simulink model "based_FOC"  (R2024b)
settings: Solver=FixedStepAuto  StartTime=0.0  StopTime=inf  FixedStep=0.000001  MaxStep=1e-6  RelTol=1e-3
undefined symbols (not defined in the file): DiscIntNeverNeededParam, F1, flux, gamma, K1, K2, L, Ld, Lq, Period, PLL_P, Pn, Rs, Ts, U_ref, Udc
libraries: eeGeneralControl x3, spsDCVoltageSourceLib x1, spsGroundLib x1, spsPermanentMagnetSynchronousMachineLib x1, slpidlib x1, simulink x1, spsTwoLevelConverterLib x1, sps_lib x1
settings Model: DataDictionary=Based_FOC_Data.sldd  SimulationMode=rapid-accelerator  Creator=sa127  LastModifiedBy=sa127
settings OptimizationCC: DefaultParameterBehavior=Inlined  UseDivisionForNetSlopeComputation=on  GainParamInheritBuiltInType=on  UseFloatMulNetSlope=on  InlineInvariantSignals=on  PassReuseOutputArgsAs=Individual arguments  ZeroExternalMemoryAtStartup=off  ZeroInternalMemoryAtStartup=off  NoFixptDivByZeroProtection=on  EfficientFloat2IntCast=on  LifeSpan=1  OptimizeBlockOrder=speed  DifferentSizesBufferReuse=on  MultiThreadedLoops=on  EfficientTunableParamExpr=on
settings DebuggingCC: ParamSuppressDoubleToSinglePrecisionLossMsg=on  ParameterTunabilityLossMsg=error
settings HardwareCC: ProdBitPerPointer=32  ProdBitPerSizeT=32  ProdBitPerPtrDiffT=32  ProdLargestAtomicInteger=Long  ProdLargestAtomicFloat=Double  ProdWordSize=32  ProdLongLongMode=on  ProdHWDeviceType=ARM Compatible->ARM Cortex-M
settings SFSimCC: MATLABDynamicMemAlloc=off
settings RTWCC: Description=Embedded Coder  SystemTargetFile=ert.tlc  TemplateMakefile=ert_default_tmf  GenerateReport=on  IncludeHyperlinkInReport=on  LaunchReport=on  GenerateTraceInfo=on  GenerateTraceReport=on  GenerateTraceReportSl=on  GenerateTraceReportSf=on  GenerateTraceReportEml=on  GenerateWebview=on  GenerateCodeMetricsReport=on  GenerateCodeReplacementReport=on
settings CodeAppCC: ForceParamTrailComments=on  IgnoreCustomStorageClasses=off  OperatorAnnotations=on  SimulinkDataObjDesc=on  SFDataObjDesc=on  CustomSymbolStrGlobalVar=rt$N$M  CustomSymbolStrType=$N$M  CustomSymbolStrFcn=$N$M$F  CustomSymbolStrMacro=$N$M  InsertBlockDesc=on
settings ERTTargetCC: TargetLangStandard=C99 (ISO)  CodeReplacementLibrary=ARM Cortex-M  GenerateSampleERTMain=on  IncludeMdlTerminateFcn=off  CombineSignalStateStructs=on  SupportComplex=off  SupportNonInlinedSFcns=on  ERTCustomFileTemplate=example_file_process.tlc  ERTFilePackagingFormat=CompactWithDataFile

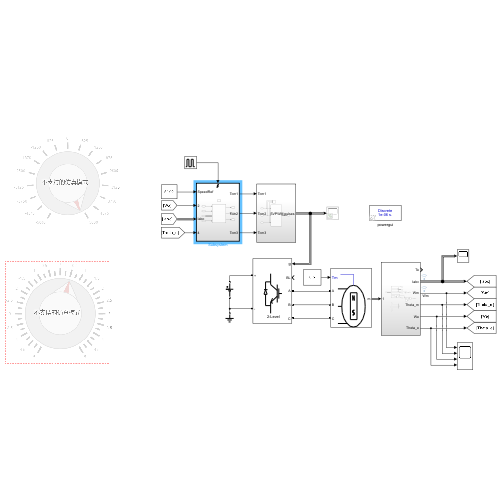
[thumbnail: Simulink's stored preview of the top-level diagram]
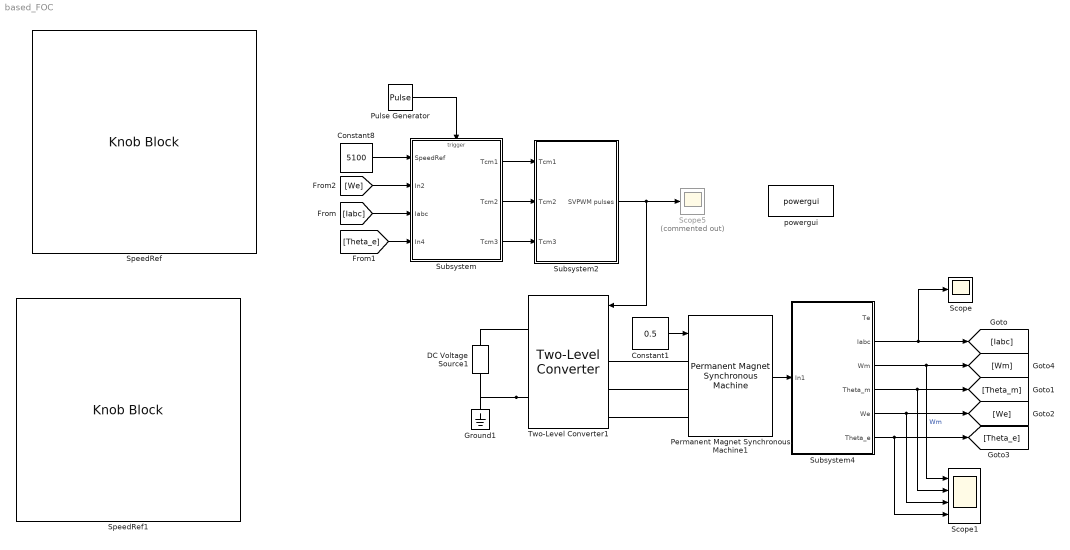
== system based_FOC ==
  Constant1 : Constant  Value=0.5
  Constant8 : Constant  Value=5100
  DC Voltage Source1 : spsDCVoltageSourceLib/DC Voltage Source  Amplitude=300  Measurements=None
  Ground1 : spsGroundLib/Ground  LConnTagsString=a
  Permanent Magnet Synchronous Machine1 : spsPermanentMagnetSynchronousMachineLib/Permanent Magnet Synchronous Machine  NbPhases=3  FluxDistribution=Sinusoidal  RotorType=Salient-pole  MechanicalLoad=Torque Tm  PresetModel="04:  6 Nm 300 Vdc 4500 RPM - 6 Nm"  ShowDetailedParameters=on  MeasurementBus=on  Resistance=0.62  Inductance=8.5e-3  dqInductances=[0.001971 0.002179]  La=0.002075  MachineConstant=Flux linkage established by magnets (V.s)  Flux=0.08627  VoltageCst=62.5906  TorqueCst=0.51762  Flat=120  Mechanical=[0.0003617 9.444e-05 4 0]  PolePairs=4  InitialConditions=[0,0, 0,0]  InitialConditions5ph=[0 0 0 0 0 0]  RefAngle=Aligned with phase A axis (original Park)  IterativeDiscreteModel=Trapezoidal non iterative  TsBlock=-1  TsPowergui=0
  Pulse Generator : DiscretePulseGenerator  PulseType=Time based  Period=0.0001  PulseWidth=50
  Scope : Scope
  Scope1 : Scope  NumInputPorts=4
  Scope5 : Scope  Commented=on
  SpeedRef : KnobBlock  ScaleMin=-5000  ScaleMax=5000
  SpeedRef1 : KnobBlock  ScaleMin=-5  ScaleMax=5
  Subsystem : Subsystem
  Subsystem2 : Subsystem
  Subsystem4 : Subsystem
  Two-Level Converter1 : spsTwoLevelConverterLib/Two-Level Converter  ModelType=Switching function  Ron=1e-3  Rs=1e6  Cs=inf  Vforward=[0,0]  Ron_Diode=1e-3  Rs_Diode=1e6  Cs_Diode=inf  Vf_Diode=1e-3  Rs_CurrentSource=inf  Ron_ACsource=1e-3
      settings: LibrarySourceBlock=sps_lib/Power Electronics/Two-Level Converter
  powergui : sps_lib/powergui  Priority=1  SimulationMode=Discrete  SampleTime=0.000001  frequency=60  Iterations=50  frequencyindice=0  Pbase=100e6  ErrMax=1e-4  UnitsV=kV  UnitsW=MW  buscounter=0  FunctionMessages=off  echomessages=off  EnableUseOfTLC=off  CurrentSourceSwitches=off  DisableSnubberDevices=off  DisableRonSwitches=off  DisableVfSwitches=off  DisplayEquations=off  AutomaticDiscreteSolvers=off  SolverType=Tustin/Backward Euler (TBE)  Interpol=off  ExternalGateDelay=off  methode=off  Ts=100  x0status=blocks  SPID=on  SwTol=0  HookPort=off  NonlinearTolerance=1e-4  nMaxIteration=100  ContinueOnMaxIteration=off  RestoreLinks=warning  ResistiveCurrentMeasurement=off  Frange=[0:2:500]  Ylog=off  Xlog=on  ShowGrid=off  save=off  variable=ZData  structure=0  ZoomFFT=off  StartTime=0.0  cycles=1  DisplayStyle=1  fundamental=60  FreqAxis=off  MaxFrequency=1000  frequencyindicesteady=1  RmsSteady=1  display=off
  wires:
  Permanent Magnet Synchronous Machine1/1 -> Subsystem4/1(In1)
  Subsystem4/2(Iabc) -> Scope/1, [Iabc]
  Subsystem4/3(Wm) -> Scope1/1, [Wm]  "Wm"
  Subsystem4/4(Theta_m) -> [Theta_m], Scope1/2
  Subsystem4/5(We) -> Scope1/3, [We]
  Subsystem4/6(Theta_e) -> Scope1/4, [Theta_e]
  Subsystem2/1(SVPWM pulses) -> Two-Level Converter1/1, Scope5/1
  Constant1/1 -> Permanent Magnet Synchronous Machine1/1
  Constant8/1 -> Subsystem/1(SpeedRef)
  [We] -> Subsystem/2(In2)
  [Iabc] -> Subsystem/3(Iabc)
  [Theta_e] -> Subsystem/4(In4)
  Subsystem/1(Tcm1) -> Subsystem2/1(Tcm1)
  Subsystem/2(Tcm2) -> Subsystem2/2(Tcm2)
  Subsystem/3(Tcm3) -> Subsystem2/3(Tcm3)
  Pulse Generator/1 -> Subsystem/Trigger
  connections:
  Two-Level Converter1/RConn2 -- DC Voltage Source1/LConn1 -- Ground1/LConn1
  Two-Level Converter1/LConn2 -- Permanent Magnet Synchronous Machine1/LConn2
  Two-Level Converter1/LConn1 -- Permanent Magnet Synchronous Machine1/LConn1
  Two-Level Converter1/LConn3 -- Permanent Magnet Synchronous Machine1/LConn3
  DC Voltage Source1/RConn1 -- Two-Level Converter1/RConn1

== system based_FOC/Subsystem ==
  SpeedRef : Inport
  In2 : Inport  Port=2
  Iabc : Inport  Port=3
  In4 : Inport  Port=4
  Trigger : TriggerPort  VariantControl=(inherit)  PortDimensions=1
  Sensorless : Subsystem
  Tcm1 : Outport
  Tcm2 : Outport  Port=2
  Tcm3 : Outport  Port=3
  wires:
  Sensorless/2(Tcm2) -> Tcm2/1
  SpeedRef/1 -> Sensorless/1(SpeedRef)
  In2/1 -> Sensorless/2(In2)
  In4/1 -> Sensorless/4(In4)
  Iabc/1 -> Sensorless/3(Iabc)
  Sensorless/3(Tcm3) -> Tcm3/1
  Sensorless/1(Tcm1) -> Tcm1/1

== system based_FOC/Subsystem2 ==
  Tcm1 : Inport
  Tcm2 : Inport  Port=2
  Tcm3 : Inport  Port=3
  Scope1 : Scope  NumInputPorts=3
  Subsystem1 : Subsystem
  SVPWM pulses : Outport
  wires:
  Tcm1/1 -> Subsystem1/1(Tcm1), Scope1/1
  Tcm2/1 -> Subsystem1/2(Tcm2), Scope1/2
  Tcm3/1 -> Subsystem1/3(Tcm3), Scope1/3
  Subsystem1/1(SVPWM pulses) -> SVPWM pulses/1

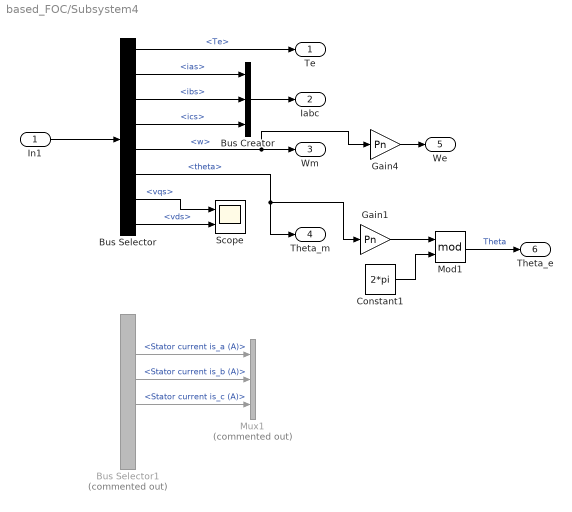
== system based_FOC/Subsystem4 ==
  In1 : Inport
  Bus Creator : BusCreator  Inputs=3
  Bus Selector : BusSelector  OutputSignals=Te,ias,ibs,ics,w,theta,vqs,vds
  Bus Selector1 : BusSelector  Commented=on  OutputSignals=Electromagnetic torque Te (N*m),Stator current is_a (A),Stator current is_b (A),Stator current is_c (A),Rotor speed wm (rad/s),Rotor angle thetam (rad)
  Constant1 : Constant  Value=2*pi
  Gain1 : Gain  Gain=Pn
  Gain4 : Gain  Gain=Pn
  Mod1 : Math  Operator=mod
  Mux1 : Mux  Commented=on  Inputs=3
  Scope : Scope  NumInputPorts=2
  Te : Outport
  Iabc : Outport  Port=2
  Wm : Outport  Port=3
  Theta_m : Outport  Port=4
  We : Outport  Port=5
  Theta_e : Outport  Port=6
  wires:
  Bus Selector/2 -> Bus Creator/1  "<ias>"
  Bus Selector/4 -> Bus Creator/3  "<ics>"
  Bus Selector/3 -> Bus Creator/2  "<ibs>"
  Bus Selector1/4 -> Mux1/3  "<Stator current is_c (A)>"
  Bus Selector1/3 -> Mux1/2  "<Stator current is_b (A)>"
  Bus Selector1/2 -> Mux1/1  "<Stator current is_a (A)>"
  In1/1 -> Bus Selector/1
  Bus Selector/1 -> Te/1  "<Te>"
  Bus Selector/5 -> Gain4/1, Wm/1  "<w>"
  Bus Selector/6 -> Gain1/1, Theta_m/1  "<theta>"
  Bus Selector/8 -> Scope/2  "<vds>"
  Bus Selector/7 -> Scope/1  "<vqs>"
  Constant1/1 -> Mod1/2
  Gain1/1 -> Mod1/1
  Gain4/1 -> We/1
  Mod1/1 -> Theta_e/1  "Theta"
  Bus Creator/1 -> Iabc/1

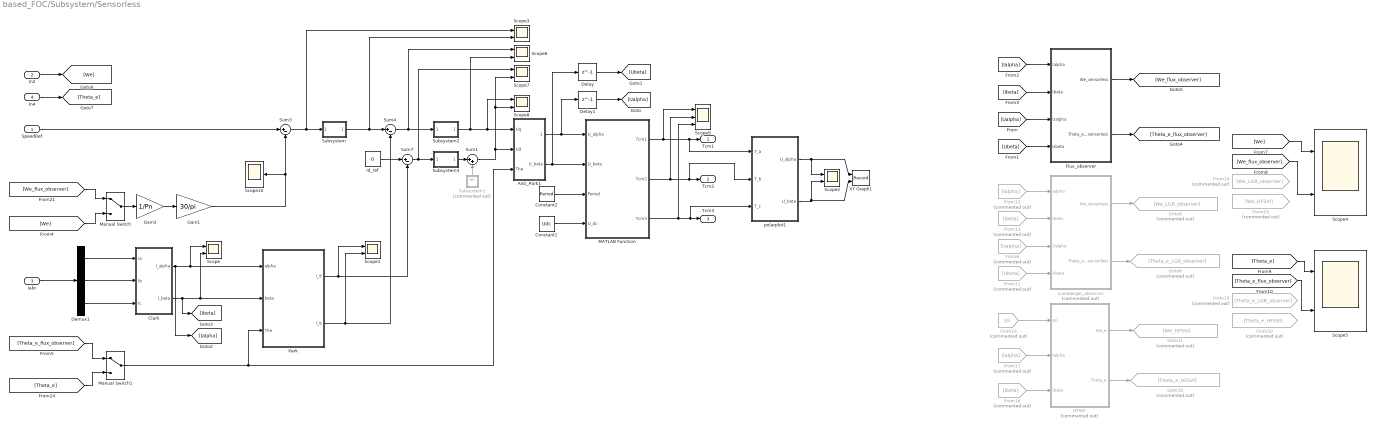
== system based_FOC/Subsystem/Sensorless ==
  SpeedRef : Inport
  In2 : Inport  Port=2
  Iabc : Inport  Port=3
  In4 : Inport  Port=4
  Anti_Park1 : Subsystem
  Clark : Subsystem
  Constant1 : Constant  Value=Udc
  Constant2 : Constant  Value=Period
  Delay : Delay  DelayLength=1
  Delay1 : Delay  DelayLength=1
  Demux1 : Demux  Outputs=3
  Flux_observer : Subsystem  TreatAsAtomicUnit=on
  From11 : From  Commented=on  GotoTag=Ubeta
  From12 : From  Commented=on  GotoTag=Ialpha
  From13 : From  Commented=on  GotoTag=Ibeta
  From14 : From  Commented=on  GotoTag=We_LGB_observer
  From15 : From  Commented=on  GotoTag=Theta_e_LGB_observer
  From16 : From  Commented=on  GotoTag=Uh  TagVisibility=global
  From17 : From  Commented=on  GotoTag=Ialpha
  From18 : From  Commented=on  GotoTag=Ibeta
  From19 : From  Commented=on  GotoTag=We_HFSVI
  From20 : From  Commented=on  GotoTag=Theta_e_HFSVI
  From6 : From  Commented=on  GotoTag=Ualpha
  Gain1 : Gain  Gain=30/pi
  Gain3 : Gain  Gain=1/Pn
  Goto10 : Goto  Commented=on  GotoTag=Theta_e_HFSVI
  Goto11 : Goto  Commented=on  GotoTag=We_HFSVI
  Goto8 : Goto  Commented=on  GotoTag=Theta_e_LGB_observer
  Goto9 : Goto  Commented=on  GotoTag=We_LGB_observer
  HFSVI : Subsystem  Commented=on
  Id_ref : Constant  Value=0
  Luenberger_observer : Subsystem  Commented=on  TreatAsAtomicUnit=on
  MATLAB Function : MATLAB Function  TreatAsAtomicUnit=on
  Manual Switch : ManualSwitch
  Manual Switch1 : ManualSwitch
  Park : Subsystem
  Scope{,1..8} (9 alike) : Scope  NumInputPorts=2
  Scope10 : Scope
  Scope9 : Scope  NumInputPorts=3
  Subsystem : Subsystem  mask{Kp=0.001, Ki=0.004, Kd=0, Ts=0.0001, max_Integral=500, min_Integral=-500, max_output=500, min_output=-500}
      mask prompts: max_Integral "积分上限"; min_Integral "积分下限"; max_output "输出上限"; min_output "输出下限"
      mask DialogControl DescTextVar Prompt: PID控制器
      mask DialogControl ParameterGroupVar Prompt: 参数
      mask Display: fprintf('MyPID');
  Subsystem1 : Subsystem  Commented=on
  Subsystem2 : Subsystem  mask{Kp=20, Ki=3000, Kd=0, Ts=0.0001, max_Integral=500, min_Integral=-500, max_output=500, min_output=-500}
      mask prompts: max_Integral "积分上限"; min_Integral "积分下限"; max_output "输出上限"; min_output "输出下限"
      mask DialogControl DescTextVar Prompt: PID控制器
      mask DialogControl ParameterGroupVar Prompt: 参数
      mask Display: fprintf('MyPID');
  Subsystem3 : Subsystem  mask{Kp=20, Ki=3000, Kd=0, Ts=0.0001, max_Integral=500, min_Integral=-500, max_output=500, min_output=-500}
      mask prompts: max_Integral "积分上限"; min_Integral "积分下限"; max_output "输出上限"; min_output "输出下限"
      mask DialogControl DescTextVar Prompt: PID控制器
      mask DialogControl ParameterGroupVar Prompt: 参数
      mask Display: fprintf('MyPID');
  Sum1 : Sum  Inputs=|++
  Sum3 : Sum  Inputs=|+-
  Sum4 : Sum  Inputs=|+-
  Sum7 : Sum  Inputs=|+-
  XY Graph1 : Record  FileSettingsInternal="{\"entries\":[{\"content\":{\"excelSettings\":{\"content\":{},\"type\":\"Streamout.ExcelSettings\"}},\"type\":\"Streamout.FileSettingStorage\",\"uuid\":\"\"}],\"packageUris\":[\"http:\\/\\/schema.mathworks.com\\/mf0\\/streamout_blocks\\/R2020a\"],\"version\":\"1.0\"}"  Layout=[1 1]  SignalsInternal="{\"entries\":[{\"content\":{\"signals\":[{\"content\":{\"blockPath\":[],\"dimensions\":[1],\"domain\":\"\",\"lineColor\":\"#ff6929\",\"plots\":[ 1 ],\"port\":1,\"sid\":[\"\"],\"signalID\":1,\"signalName\":\"polarplot1:1\"},\"type\":\"RecordBlkView.Signal\",\"uuid\":\"\"},{\"content\":{\"blockPath\":[],\"dimensions\":[1],\"domain\":\"\",\"lineColor\":\"#b746ff\",\"plots\":[ 1 ],\"port\":2,\"sid\":[\"\"],\"signalID\":2,\"signalName\":\"polarplot1:2\"},\"type\":\"RecordBlkView.Signal\",\"uuid\":\"\"}]},\"type\":\"RecordBlkView.InputSignals\",\"uuid\":\"\"}],\"packageUris\":[\"http:\\/\\/schema.mathworks.com\\/mf0\\/streamout_blocks\\/R2020a\"],\"version\":\"1.0\"}"  VisualizationBindings="{\"xyplotplugin\":{\"info\":[{\"series\":[{\"bindingParametersList\":[{\"parameter\":\"X-Axis\",\"signalID\":1,\"signalName\":\"polarplot1:1\"},{\"parameter\":\"Y-Axis\",\"signalID\":2,\"signalName\":\"polarplot1:2\"},{\"parameter\":\"X-Axis\",\"signalID\":1,\"signalName\":\"polarplot1:1\"},{\"parameter\":\"Y-Axis\",\"signalID\":2,\"signalName\":\"polarplot1:2\"}],\"seriesID\":0}],\"subplotID\":1}]}}"  CompatibilityTag=XY
  polarplot1 : MATLAB Function  TreatAsAtomicUnit=on
  Tcm1 : Outport
  Tcm2 : Outport  Port=2
  Tcm3 : Outport  Port=3
  wires:
  Park/1(I_d) -> Scope1/1, Sum7/2
  Sum7/1 -> Scope7/1, Subsystem3/1(error)
  Gain1/1 -> Sum3/2, Scope10/1
  Demux1/3 -> Clark/3(Ic)
  Demux1/1 -> Clark/1(Ia)
  Iabc/1 -> Demux1/1
  Clark/1(I_alpha) -> [Ialpha], Scope/1, Park/1(alpha)
  Clark/2(I_beta) -> [Ibeta], Scope/2, Park/2(beta)
  Id_ref/1 -> Sum7/1
  Sum3/1 -> Scope3/1, Subsystem/1(error)
  Park/2(I_q) -> Scope1/2, Sum4/2
  Sum4/1 -> Scope6/1, Subsystem2/1(error)
  Demux1/2 -> Clark/2(Ib)
  Gain3/1 -> Gain1/1
  SpeedRef/1 -> Sum3/1
  Anti_Park1/2(U_beta) -> MATLAB Function/2(U_beta), Delay/1
  Subsystem2/1(output) -> Scope6/2, Anti_Park1/1(Uq), Scope8/1
  Manual Switch1/1 -> Anti_Park1/3(The), Park/3(The)
  [We] -> Scope4/1
  [Theta_e] -> Scope5/1
  Delay/1 -> [Ubeta]
  Delay1/1 -> [Ualpha]
  [Ialpha] -> Flux_observer/1(Ialpha)
  [Ibeta] -> Flux_observer/2(Ibeta)
  [Ualpha] -> Flux_observer/3(Ualpha)
  [Ubeta] -> Flux_observer/4(Ubeta)
  Flux_observer/2(Theta_e_sensorless) -> [Theta_e_flux_observer]
  Flux_observer/1(We_sensorless) -> [We_flux_observer]
  In2/1 -> [We]
  In4/1 -> [Theta_e]
  From12/1 -> Luenberger_observer/1(Ialpha)
  From13/1 -> Luenberger_observer/2(Ibeta)
  From6/1 -> Luenberger_observer/3(Ualpha)
  From11/1 -> Luenberger_observer/4(Ubeta)
  Luenberger_observer/1(We_sensorless) -> Goto9/1
  Luenberger_observer/2(Theta_e_sensorless) -> Goto8/1
  Subsystem/1(output) -> Scope3/2, Sum4/1
  Subsystem3/1(output) -> Sum1/1
  Sum1/1 -> Anti_Park1/2(Ud), Scope8/2, Scope7/2
  From16/1 -> HFSVI/1(Uh)
  From17/1 -> HFSVI/2(Ialpha)
  From18/1 -> HFSVI/3(Ibeta)
  HFSVI/2(Theta_e) -> Goto10/1
  HFSVI/1(We_e) -> Goto11/1
  Manual Switch/1 -> Gain3/1
  [We] -> Manual Switch/2
  [We_flux_observer] -> Manual Switch/1
  [Theta_e] -> Manual Switch1/2
  [Theta_e_flux_observer] -> Manual Switch1/1
  Subsystem1/1(Uh) -> Sum1/2
  [We_flux_observer] -> Scope4/2
  [Theta_e_flux_observer] -> Scope5/2
  Anti_Park1/1(U_alpha) -> MATLAB Function/1(U_alpha), Delay1/1
  Constant2/1 -> MATLAB Function/3(Period)
  Constant1/1 -> MATLAB Function/4(U_dc)
  MATLAB Function/1(Tcm1) -> polarplot1/1(T_a), Tcm1/1, Scope9/1
  MATLAB Function/2(Tcm2) -> polarplot1/2(T_b), Tcm2/1, Scope9/2
  MATLAB Function/3(Tcm3) -> polarplot1/3(T_c), Tcm3/1, Scope9/3
  polarplot1/1(U_alpha) -> XY Graph1/1, Scope2/1
  polarplot1/2(U_beta) -> XY Graph1/2, Scope2/2

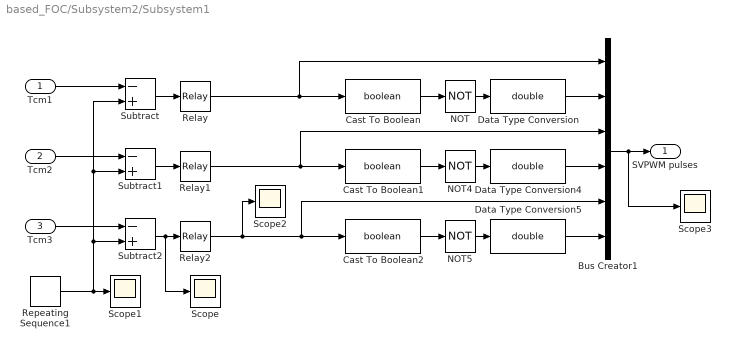
== system based_FOC/Subsystem2/Subsystem1 ==
  Tcm1 : Inport
  Tcm2 : Inport  Port=2
  Tcm3 : Inport  Port=3
  Bus Creator1 : BusCreator  Inputs=6
  Cast To Boolean : DataTypeConversion  OutDataTypeStr=boolean  SaturateOnIntegerOverflow=off  RndMeth=Floor
  Cast To Boolean1 : DataTypeConversion  OutDataTypeStr=boolean  SaturateOnIntegerOverflow=off  RndMeth=Floor
  Cast To Boolean2 : DataTypeConversion  OutDataTypeStr=boolean  SaturateOnIntegerOverflow=off  RndMeth=Floor
  Data Type Conversion : DataTypeConversion  OutDataTypeStr=double  SaturateOnIntegerOverflow=off  RndMeth=Floor
  Data Type Conversion4 : DataTypeConversion  OutDataTypeStr=double  SaturateOnIntegerOverflow=off  RndMeth=Floor
  Data Type Conversion5 : DataTypeConversion  OutDataTypeStr=double  SaturateOnIntegerOverflow=off  RndMeth=Floor
  NOT : Logic  Operator=NOT  IconShape=distinctive  AllPortsSameDT=off  OutDataTypeStr=boolean
  NOT4 : Logic  Operator=NOT  IconShape=distinctive  AllPortsSameDT=off  OutDataTypeStr=boolean
  NOT5 : Logic  Operator=NOT  IconShape=distinctive  AllPortsSameDT=off  OutDataTypeStr=boolean
  Relay : Relay
  Relay1 : Relay
  Relay2 : Relay
  Repeating Sequence1 : simulink/Sources/Repeating Sequence  rep_seq_t=[0 Ts/2 Ts]  rep_seq_y=[0 Period/2 0]
  Scope{,1..3} (4 alike) : Scope
  Subtract : Sum  Inputs=-+
  Subtract1 : Sum  Inputs=-+
  Subtract2 : Sum  Inputs=-+
  SVPWM pulses : Outport
  wires:
  Tcm3/1 -> Subtract2/1
  Cast To Boolean/1 -> NOT/1
  Subtract/1 -> Relay/1
  Relay2/1 -> Scope2/1, Bus Creator1/5, Cast To Boolean2/1
  Subtract2/1 -> Scope/1, Relay2/1
  Cast To Boolean2/1 -> NOT5/1
  Subtract1/1 -> Relay1/1
  Repeating Sequence1/1 -> Subtract2/2, Subtract1/2, Subtract/2, Scope1/1
  Tcm1/1 -> Subtract/1
  NOT/1 -> Data Type Conversion/1
  Cast To Boolean1/1 -> NOT4/1
  Bus Creator1/1 -> Scope3/1, SVPWM pulses/1
  NOT5/1 -> Data Type Conversion5/1
  Relay1/1 -> Bus Creator1/3, Cast To Boolean1/1
  Relay/1 -> Bus Creator1/1, Cast To Boolean/1
  Tcm2/1 -> Subtract1/1
  Data Type Conversion5/1 -> Bus Creator1/6
  Data Type Conversion/1 -> Bus Creator1/2
  NOT4/1 -> Data Type Conversion4/1
  Data Type Conversion4/1 -> Bus Creator1/4

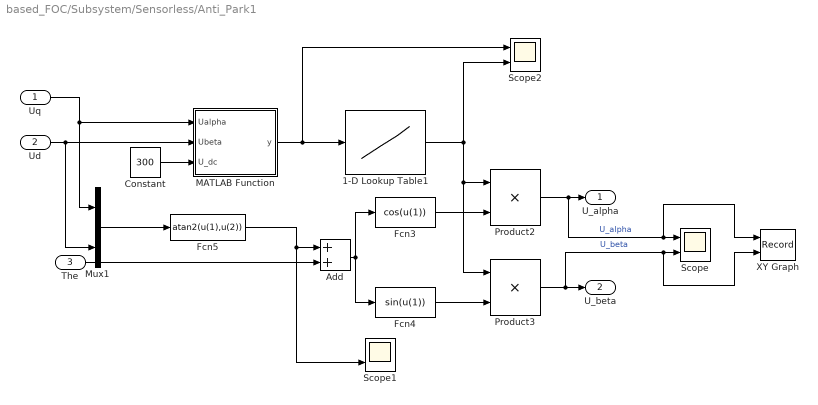
== system based_FOC/Subsystem/Sensorless/Anti_Park1 ==
  Uq : Inport
  Ud : Inport  Port=2
  The : Inport  Port=3
  1-D Lookup Table1 : Lookup_n-D  NumberOfTableDimensions=1  BreakpointsForDimension1=F1  Table=U_ref  ExtrapMethod=Clip  UseLastTableValue=on  InternalRulePriority=Speed  RndMeth=Simplest
  Add : Sum
  Constant : Constant  Value=300
  Fcn3 : Fcn  Expr=cos(u(1))
  Fcn4 : Fcn  Expr=sin(u(1))
  Fcn5 : Fcn  Expr=atan2(u(1),u(2))
  MATLAB Function : MATLAB Function  TreatAsAtomicUnit=on
  Mux1 : Mux  Inputs=2
  Product2 : Product
  Product3 : Product
  Scope : Scope  NumInputPorts=2
  Scope1 : Scope  NumInputPorts=2
  Scope2 : Scope  NumInputPorts=2
  XY Graph : Record  FileSettingsInternal="{\"entries\":[{\"content\":{\"excelSettings\":{\"content\":{},\"type\":\"Streamout.ExcelSettings\"}},\"type\":\"Streamout.FileSettingStorage\",\"uuid\":\"\"}],\"packageUris\":[\"http:\\/\\/schema.mathworks.com\\/mf0\\/streamout_blocks\\/R2020a\"],\"version\":\"1.0\"}"  Layout=[1 1]  SignalsInternal="{\"entries\":[{\"content\":{\"signals\":[{\"content\":{\"blockPath\":[],\"dimensions\":[1],\"domain\":\"\",\"lineColor\":\"#139fff\",\"lineWidth\":2,\"plots\":[ 1 ],\"port\":1,\"sid\":[\"\"],\"signalID\":1,\"signalName\":\"U_alpha\"},\"type\":\"RecordBlkView.Signal\",\"uuid\":\"\"},{\"content\":{\"blockPath\":[],\"dimensions\":[1],\"domain\":\"\",\"lineColor\":\"#22b573\",\"lineWidth\":2,\"plots\":[ 1 ],\"port\":2,\"sid\":[\"\"],\"signalID\":2,\"signalName\":\"U_beta\"},\"type\":\"RecordBlkView.Signal\",\"uuid\":\"\"}]},\"type\":\"RecordBlkView.InputSignals\",\"uuid\":\"\"}],\"packageUris\":[\"http:\\/\\/schema.mathworks.com\\/mf0\\/streamout_blocks\\/R2020a\"],\"version\":\"1.0\"}"  VisualizationBindings="{\"xyplotplugin\":{\"info\":[{\"series\":[{\"bindingParametersList\":[{\"parameter\":\"X-Axis\",\"signalID\":1,\"signalName\":\"U_alpha\"},{\"parameter\":\"Y-Axis\",\"signalID\":2,\"signalName\":\"U_beta\"},{\"parameter\":\"X-Axis\",\"signalID\":1,\"signalName\":\"U_alpha\"},{\"parameter\":\"Y-Axis\",\"signalID\":2,\"signalName\":\"U_beta\"}],\"seriesID\":0}],\"subplotID\":1}]}}"  CompatibilityTag=XY
  U_alpha : Outport
  U_beta : Outport  Port=2
  wires:
  Fcn5/1 -> Scope1/2, Add/1
  Ud/1 -> MATLAB Function/2(Ubeta), Mux1/2
  Fcn3/1 -> Product2/2
  Fcn4/1 -> Product3/2
  Mux1/1 -> Fcn5/1
  1-D Lookup Table1/1 -> Scope2/2, Product2/1, Product3/1
  Product2/1 -> XY Graph/1, Scope/1, U_alpha/1  "U_alpha"
  Product3/1 -> XY Graph/2, Scope/2, U_beta/1  "U_beta"
  The/1 -> Add/2
  Add/1 -> Fcn3/1, Fcn4/1
  Constant/1 -> MATLAB Function/3(U_dc)
  Uq/1 -> MATLAB Function/1(Ualpha), Mux1/1
  MATLAB Function/1(y) -> 1-D Lookup Table1/1, Scope2/1

== system based_FOC/Subsystem/Sensorless/Clark ==
  Ia : Inport
  Ib : Inport  Port=2
  Ic : Inport  Port=3
  Fcn : Fcn  Expr=(u(1)-0.5*u(2)-0.5*u(3))*2/3
  Fcn1 : Fcn  Expr=(sqrt(3)/2*u(2)-sqrt(3)/2*u(3))*2/3
  Mux : Mux  Inputs=3
  I_alpha : Outport
  I_beta : Outport  Port=2
  wires:
  Ib/1 -> Mux/2
  Fcn1/1 -> I_beta/1
  Ic/1 -> Mux/3
  Mux/1 -> Fcn1/1, Fcn/1
  Fcn/1 -> I_alpha/1
  Ia/1 -> Mux/1

== system based_FOC/Subsystem/Sensorless/Flux_observer ==
  Ialpha : Inport
  Ibeta : Inport  Port=2
  Ualpha : Inport  Port=3
  Ubeta : Inport  Port=4
  OBSERVER : Subsystem
  PLL : Subsystem
  Scope : Scope  NumInputPorts=2
  We_sensorless : Outport
  Theta_e_sensorless : Outport  Port=2
  wires:
  Ibeta/1 -> OBSERVER/2(Ibeta)
  OBSERVER/1(sin) -> Scope/1, PLL/1(sin)  "sin_theta"
  OBSERVER/2(cos) -> Scope/2, PLL/2(cos)  "cos_theta"
  PLL/1(We) -> We_sensorless/1
  PLL/2(Theta_e) -> Theta_e_sensorless/1
  Ualpha/1 -> OBSERVER/3(Ualpha)
  Ubeta/1 -> OBSERVER/4(Ubeta)
  Ialpha/1 -> OBSERVER/1(Ialpha)

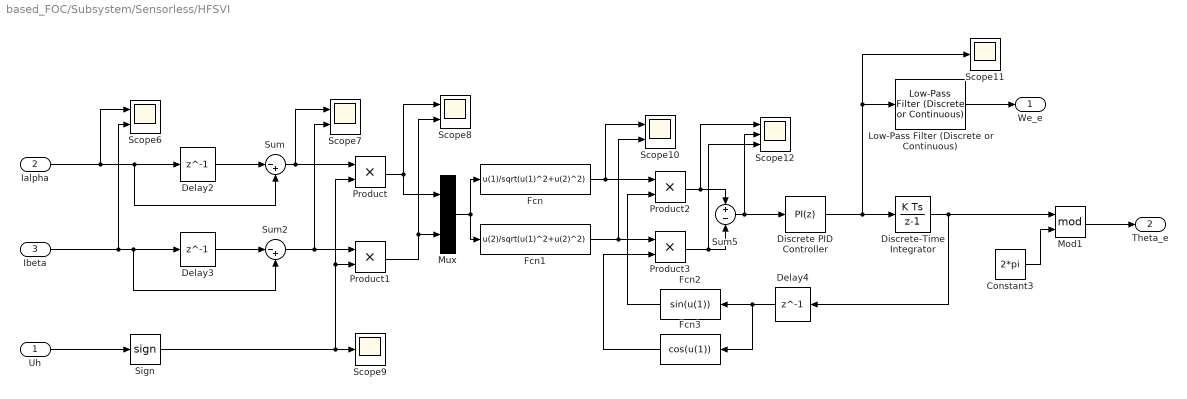
== system based_FOC/Subsystem/Sensorless/HFSVI ==
  Uh : Inport
  Ialpha : Inport  Port=2
  Ibeta : Inport  Port=3
  Constant3 : Constant  Value=2*pi
  Delay2 : Delay  DelayLength=1  InitialCondition=0
  Delay3 : Delay  DelayLength=1  InitialCondition=0
  Delay4 : Delay  DelayLength=1  InitialCondition=0
  Discrete PID Controller : slpidlib/PID Controller  Controller=PI  Form=Parallel  TimeDomain=Discrete-time  UseExternalTs=off  SampleTime=-1  IntegratorMethod=Forward Euler  FilterMethod=Forward Euler  ControllerParametersSource=internal  P=400  I=40000  UseKiTs=off  D=0  UseExternalDerivativeSource=off  N=100  UseFilter=on  TunerSelectOption=Transfer Function Based (PID Tuner App)  InitialConditionSource=internal  InitialConditionForIntegrator=0  InitialConditionForFilter=0  DifferentiatorICPrevScaledInput=0  ExternalReset=none  TrackingMode=off  Kt=1  LimitOutput=off  SatLimitsSource=internal  UpperSaturationLimit=inf  LowerSaturationLimit=-inf  LinearizeAsGain=off  AntiWindupMode=none  Kb=1  LimitIntegrator=off  UpperIntegratorSaturationLimit=inf  LowerIntegratorSaturationLimit=-inf  POutMin=[]  POutMax=[]  IOutMin=[]  IOutMax=[]  DOutMin=[]  DOutMax=[]  NOutMin=[]  NOutMax=[]  SumOutMin=[]  SumOutMax=[]  SaturationOutMin=[]  SaturationOutMax=[]  PParamMin=[]  PParamMax=[]  IParamMin=[]  IParamMax=[]  DParamMin=[]  DParamMax=[]  NParamMin=[]  NParamMax=[]  KbParamMin=[]  KbParamMax=[]  KtParamMin=[]  KtParamMax=[]  KbOutMin=[]  KbOutMax=[]  KtOutMin=[]  KtOutMax=[]  IntegratorOutMin=[]  IntegratorOutMax=[]  FilterOutMin=[]  FilterOutMax=[]  SumI1OutMin=[]  SumI1OutMax=[]  SumI2OutMin=[]  SumI2OutMax=[]  SumI3OutMin=[]  SumI3OutMax=[]  SumI4OutMin=[]  SumI4OutMax=[]  SumDOutMin=[]  SumDOutMax=[]  DifferentiatorOutMin=[]  DifferentiatorOutMax=[]  FilterDiffOutCoefMin=[]  FilterDiffOutCoefMax=[]  ReciprocalOutMin=[]  ReciprocalOutMax=[]  SumDenOutMin=[]  SumDenOutMax=[]  SumNumOutMin=[]  SumNumOutMax=[]  DivideOutMin=[]  DivideOutMax=[]  UdiffTsProdOutMin=[]  UdiffTsProdOutMax=[]  NTsProdOutMin=[]  NTsProdOutMax=[]  UintegralTsProdOutMin=[]  UintegralTsProdOutMax=[]  UngainTsProdOutMin=[]  UngainTsProdOutMax=[]  ClampingZeroOutDataTypeStr=Inherit: Inherit via back propagation  ClampingZeroOutMin=[]  ClampingZeroOutMax=[]  FilterDenConstantOutDataTypeStr=Inherit: Inherit via back propagation  FilterDenConstantOutMin=[]  FilterDenConstantOutMax=[]  PCopyOutDataTypeStr=Inherit: Inherit via back propagation  PCopyOutMin=[]  PCopyOutMax=[]  NCopyOutDataTypeStr=Inherit: Inherit via back propagation  NCopyOutMin=[]  NCopyOutMax=[]  IntegratorContinuousStateAttributes=''  IntegratorStateMustResolveToSignalObject=off  IntegratorRTWStateStorageClass=Auto  FilterContinuousStateAttributes=''  FilterStateMustResolveToSignalObject=off  FilterRTWStateStorageClass=Auto  ParallelPVariant=InternalParameters  IdealPVariant=Disabled  IVariant=InternalParameters  DVariant=Disabled  IntegratorVariant=Discrete  SatVariant=Disabled  AWVariant=Passthrough  PCopyVariant=Disabled  TRVariant=Disabled  FdbkBlocksVariant=Forward  IdealPFdbkVariant=Disabled  SatFdbkVariant=Disabled  DerivativeFilterVariant=Disabled  NVariant=Disabled  NCopyVariant=Disabled_SignalSpec  FilterICVariant=Disabled  IntegratorICVariant=InternalICs  ExternalResetVariant=Disabled  TRSumVariant=Passthrough  SumFdbkVariant=Disabled  SumVariant=Sum_PI  TsampFilterVariant=InternalTs  TsampNgainVariant=Passthrough  TsampIntegralVariant=Disabled_SignalSpec  ExternalSaturationOutDataTypeStr=Inherit: Same as second input  DerivativeSourceVariant=Disabled  PreIntVariant=InternalPreInt
  Discrete-Time Integrator : DiscreteIntegrator  SampleTime=-1  ICPrevOutput=DiscIntNeverNeededParam  ICPrevScaledInput=DiscIntNeverNeededParam
  Fcn : Fcn  Expr=u(1)/sqrt(u(1)^2+u(2)^2)
  Fcn1 : Fcn  Expr=u(2)/sqrt(u(1)^2+u(2)^2)
  Fcn2 : Fcn  Expr=sin(u(1))
  Fcn3 : Fcn  Expr=cos(u(1))
  Low-Pass Filter (Discrete or Continuous) : eeGeneralControl/Low-Pass Filter (Discrete or Continuous)  K=1  T=0.02  B=inf  A=-inf  init_option=Inherited from block input  x0=0  Ts=-1
  Mod1 : Math  Operator=mod
  Mux : Mux  Inputs=2
  Product{,1..3} (4 alike) : Product
  Scope{6..8,10} (4 alike) : Scope  NumInputPorts=2
  Scope11 : Scope
  Scope12 : Scope  NumInputPorts=3
  Scope9 : Scope
  Sign : Signum
  Sum : Sum  Inputs=|-+
  Sum2 : Sum  Inputs=|-+
  Sum5 : Sum  Inputs=+-
  We_e : Outport
  Theta_e : Outport  Port=2
  wires:
  Sum2/1 -> Scope7/2, Product1/1
  Ibeta/1 -> Delay3/1, Sum2/2, Scope6/2
  Discrete-Time Integrator/1 -> Delay4/1, Mod1/1
  Product2/1 -> Sum5/1, Scope12/1
  Discrete PID Controller/1 -> Discrete-Time Integrator/1, Scope11/1, Low-Pass Filter (Discrete or Continuous)/1
  Uh/1 -> Sign/1
  Fcn1/1 -> Product3/1, Scope10/2
  Mux/1 -> Fcn/1, Fcn1/1
  Product/1 -> Scope8/1, Mux/1
  Sum/1 -> Scope7/1, Product/1
  Product3/1 -> Scope12/3, Sum5/2
  Delay4/1 -> Fcn2/1, Fcn3/1
  Product1/1 -> Scope8/2, Mux/2
  Ialpha/1 -> Scope6/1, Delay2/1, Sum/2
  Low-Pass Filter (Discrete or Continuous)/1 -> We_e/1
  Delay3/1 -> Sum2/1
  Sum5/1 -> Discrete PID Controller/1, Scope12/2
  Sign/1 -> Product/2, Product1/2, Scope9/1
  Delay2/1 -> Sum/1
  Fcn2/1 -> Product2/2
  Fcn3/1 -> Product3/2
  Fcn/1 -> Scope10/1, Product2/1
  Constant3/1 -> Mod1/2
  Mod1/1 -> Theta_e/1

== system based_FOC/Subsystem/Sensorless/Luenberger_observer ==
  Ialpha : Inport
  Ibeta : Inport  Port=2
  Ualpha : Inport  Port=3
  Ubeta : Inport  Port=4
  OBSERVER : Subsystem
  PLL : Subsystem
  Scope6 : Scope  NumInputPorts=2
  We_sensorless : Outport
  Theta_e_sensorless : Outport  Port=2
  wires:
  Ibeta/1 -> OBSERVER/2(Ibeta)
  OBSERVER/1(Ealpha_hat) -> PLL/1(Ealpha_hat), Scope6/1  "sin_theta"
  OBSERVER/2(Ebeta_hat) -> PLL/2(Ebeta_hat), Scope6/2  "cos_theta"
  PLL/1(We) -> We_sensorless/1, OBSERVER/5(We)
  PLL/2(Theta_e) -> Theta_e_sensorless/1
  Ualpha/1 -> OBSERVER/3(Ualpha)
  Ubeta/1 -> OBSERVER/4(Ubeta)
  Ialpha/1 -> OBSERVER/1(Ialpha)

== system based_FOC/Subsystem/Sensorless/Park ==
  alpha : Inport
  beta : Inport  Port=2
  The : Inport  Port=3
  Fcn : Fcn  Expr=cos(u(3))*u(1)+sin(u(3))*u(2)
  Fcn1 : Fcn  Expr=-sin(u(3))*u(1)+cos(u(3))*u(2)
  Mux : Mux  Inputs=3
  I_d : Outport
  I_q : Outport  Port=2
  wires:
  Fcn/1 -> I_d/1
  Fcn1/1 -> I_q/1
  The/1 -> Mux/3
  alpha/1 -> Mux/1
  Mux/1 -> Fcn1/1, Fcn/1
  beta/1 -> Mux/2

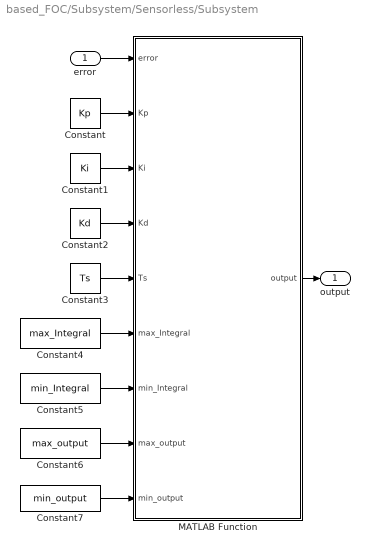
== system based_FOC/Subsystem/Sensorless/Subsystem ==
  error : Inport
  Constant : Constant  Value=Kp
  Constant1 : Constant  Value=Ki
  Constant2 : Constant  Value=Kd
  Constant3 : Constant  Value=Ts
  Constant4 : Constant  Value=max_Integral
  Constant5 : Constant  Value=min_Integral
  Constant6 : Constant  Value=max_output
  Constant7 : Constant  Value=min_output
  MATLAB Function : MATLAB Function  TreatAsAtomicUnit=on
  output : Outport
  wires:
  Constant3/1 -> MATLAB Function/5(Ts)
  Constant7/1 -> MATLAB Function/9(min_output)
  Constant/1 -> MATLAB Function/2(Kp)
  Constant4/1 -> MATLAB Function/6(max_Integral)
  Constant5/1 -> MATLAB Function/7(min_Integral)
  error/1 -> MATLAB Function/1(error)
  Constant1/1 -> MATLAB Function/3(Ki)
  Constant6/1 -> MATLAB Function/8(max_output)
  Constant2/1 -> MATLAB Function/4(Kd)
  MATLAB Function/1(output) -> output/1

== system based_FOC/Subsystem/Sensorless/Subsystem1 ==
  MATLAB Function : MATLAB Function  TreatAsAtomicUnit=on
  Scope1 : Scope
  Uh : Outport
  tag scope: Uh=global
  wires:
  MATLAB Function/1(y) -> [Uh], Uh/1, Scope1/1

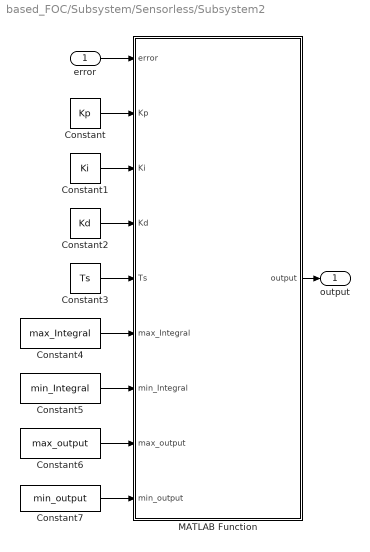
== system based_FOC/Subsystem/Sensorless/Subsystem2 ==
  error : Inport
  Constant : Constant  Value=Kp
  Constant1 : Constant  Value=Ki
  Constant2 : Constant  Value=Kd
  Constant3 : Constant  Value=Ts
  Constant4 : Constant  Value=max_Integral
  Constant5 : Constant  Value=min_Integral
  Constant6 : Constant  Value=max_output
  Constant7 : Constant  Value=min_output
  MATLAB Function : MATLAB Function  TreatAsAtomicUnit=on
  output : Outport
  wires:
  MATLAB Function/1(output) -> output/1
  Constant2/1 -> MATLAB Function/4(Kd)
  Constant6/1 -> MATLAB Function/8(max_output)
  Constant1/1 -> MATLAB Function/3(Ki)
  error/1 -> MATLAB Function/1(error)
  Constant5/1 -> MATLAB Function/7(min_Integral)
  Constant4/1 -> MATLAB Function/6(max_Integral)
  Constant/1 -> MATLAB Function/2(Kp)
  Constant7/1 -> MATLAB Function/9(min_output)
  Constant3/1 -> MATLAB Function/5(Ts)

== system based_FOC/Subsystem/Sensorless/Subsystem3 ==
  error : Inport
  Constant : Constant  Value=Kp
  Constant1 : Constant  Value=Ki
  Constant2 : Constant  Value=Kd
  Constant3 : Constant  Value=Ts
  Constant4 : Constant  Value=max_Integral
  Constant5 : Constant  Value=min_Integral
  Constant6 : Constant  Value=max_output
  Constant7 : Constant  Value=min_output
  MATLAB Function : MATLAB Function  TreatAsAtomicUnit=on
  output : Outport
  wires:
  Constant3/1 -> MATLAB Function/5(Ts)
  Constant7/1 -> MATLAB Function/9(min_output)
  Constant/1 -> MATLAB Function/2(Kp)
  Constant4/1 -> MATLAB Function/6(max_Integral)
  Constant5/1 -> MATLAB Function/7(min_Integral)
  error/1 -> MATLAB Function/1(error)
  Constant1/1 -> MATLAB Function/3(Ki)
  Constant6/1 -> MATLAB Function/8(max_output)
  Constant2/1 -> MATLAB Function/4(Kd)
  MATLAB Function/1(output) -> output/1

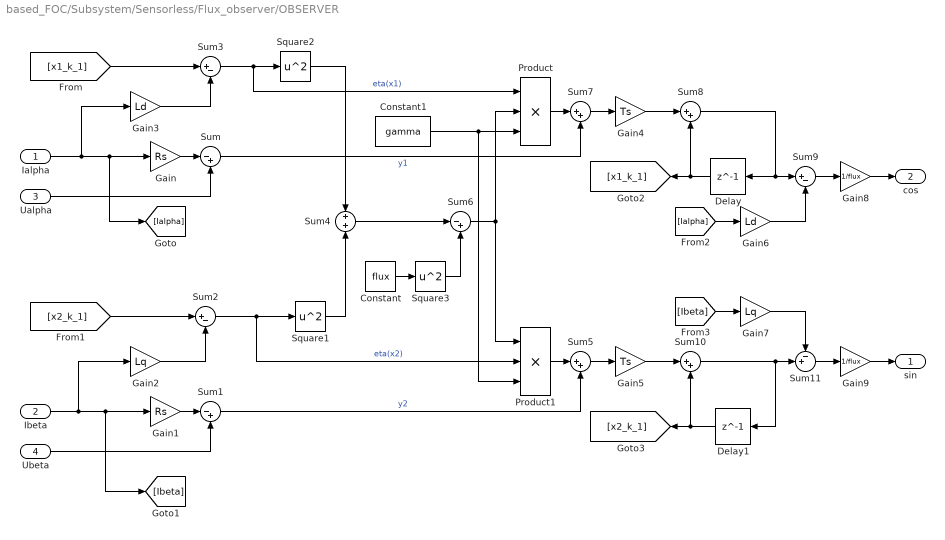
== system based_FOC/Subsystem/Sensorless/Flux_observer/OBSERVER ==
  Ialpha : Inport
  Ibeta : Inport  Port=2
  Ualpha : Inport  Port=3
  Ubeta : Inport  Port=4
  Constant : Constant  Value=flux
  Constant1 : Constant  Value=gamma
  Delay : Delay  DelayLength=1  InputProcessing=Columns as channels (frame based)
  Delay1 : Delay  DelayLength=1  InputProcessing=Columns as channels (frame based)
  Gain : Gain  Gain=Rs
  Gain1 : Gain  Gain=Rs
  Gain2 : Gain  Gain=Lq
  Gain3 : Gain  Gain=Ld
  Gain4 : Gain  Gain=Ts
  Gain5 : Gain  Gain=Ts
  Gain6 : Gain  Gain=Ld
  Gain7 : Gain  Gain=Lq
  Gain8 : Gain  Gain=1/flux
  Gain9 : Gain  Gain=1/flux
  Product : Product  Inputs=3
  Product1 : Product  Inputs=3
  Square1 : Math  Operator=square
  Square2 : Math  Operator=square
  Square3 : Math  Operator=square
  Sum : Sum  Inputs=|-+
  Sum1 : Sum  Inputs=|-+
  Sum{5,7..8,10} (4 alike) : Sum  Inputs=|++
  Sum11 : Sum  Inputs=-+|
  Sum2 : Sum  Inputs=|+-
  Sum3 : Sum  Inputs=|+-
  Sum4 : Sum
  Sum6 : Sum  Inputs=|-+
  Sum9 : Sum  Inputs=|+-
  sin : Outport
  cos : Outport  Port=2
  wires:
  Ialpha/1 -> Gain3/1, [Ialpha], Gain/1
  Gain/1 -> Sum/1
  Ualpha/1 -> Sum/2
  Ubeta/1 -> Sum1/2
  Gain1/1 -> Sum1/1
  Ibeta/1 -> Gain2/1, [Ibeta], Gain1/1
  Sum1/1 -> Sum5/2  "y2"
  Sum/1 -> Sum7/2  "y1"
  [x2_k_1] -> Sum2/1
  [x1_k_1] -> Sum3/1
  Gain2/1 -> Sum2/2
  Gain3/1 -> Sum3/2
  Sum3/1 -> Product/1, Square2/1  "eta(x1)"
  Sum2/1 -> Product1/2, Square1/1  "eta(x2)"
  Square2/1 -> Sum4/1
  Square1/1 -> Sum4/2
  Sum4/1 -> Sum6/1
  Square3/1 -> Sum6/2
  Constant/1 -> Square3/1
  Sum6/1 -> Product1/1, Product/2
  Constant1/1 -> Product1/3, Product/3
  Product1/1 -> Sum5/1
  Product/1 -> Sum7/1
  Sum5/1 -> Gain5/1
  Sum7/1 -> Gain4/1
  Sum8/1 -> Sum9/1, Delay/1
  Delay/1 -> [x1_k_1], Sum8/2
  Gain4/1 -> Sum8/1
  Sum10/1 -> Sum11/2, Delay1/1
  Delay1/1 -> [x2_k_1], Sum10/2
  Gain5/1 -> Sum10/1
  [Ialpha] -> Gain6/1
  [Ibeta] -> Gain7/1
  Gain6/1 -> Sum9/2
  Gain7/1 -> Sum11/1
  Sum9/1 -> Gain8/1
  Gain8/1 -> cos/1
  Gain9/1 -> sin/1
  Sum11/1 -> Gain9/1

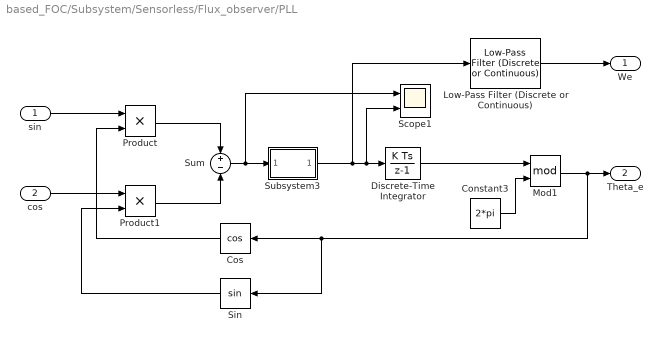
== system based_FOC/Subsystem/Sensorless/Flux_observer/PLL ==
  sin : Inport
  cos : Inport  Port=2
  Constant3 : Constant  Value=2*pi
  Cos : Trigonometry  Operator=cos  ApproximationMethod=Lookup
  Discrete-Time Integrator : DiscreteIntegrator  SampleTime=-1  ICPrevOutput=DiscIntNeverNeededParam  ICPrevScaledInput=DiscIntNeverNeededParam
  Low-Pass Filter (Discrete or Continuous) : eeGeneralControl/Low-Pass Filter (Discrete or Continuous)  K=1  T=0.01  B=inf  A=-inf  init_option=Inherited from block input  x0=0  Ts=-1
  Mod1 : Math  Operator=mod
  Product : Product
  Product1 : Product
  Scope1 : Scope  NumInputPorts=2
  Sin : Trigonometry  ApproximationMethod=Lookup
  Subsystem3 : Subsystem  mask{Kp=PLL_P, Ki=30000, Kd=0, Ts=0.0001, max_Integral=Inf, min_Integral=-Inf, max_output=inf, min_output=-inf}
      mask prompts: max_Integral "积分上限"; min_Integral "积分下限"; max_output "输出上限"; min_output "输出下限"
      mask DialogControl DescTextVar Prompt: PID控制器
      mask DialogControl ParameterGroupVar Prompt: 参数
      mask Display: fprintf('MyPID');
  Sum : Sum  Inputs=+-
  We : Outport
  Theta_e : Outport  Port=2
  wires:
  Mod1/1 -> Sin/1, Cos/1, Theta_e/1
  Constant3/1 -> Mod1/2
  Subsystem3/1(output) -> Low-Pass Filter (Discrete or Continuous)/1, Scope1/2, Discrete-Time Integrator/1
  Sin/1 -> Product1/2
  Cos/1 -> Product/2
  Product/1 -> Sum/1
  Product1/1 -> Sum/2
  Discrete-Time Integrator/1 -> Mod1/1
  Sum/1 -> Subsystem3/1(error), Scope1/1
  sin/1 -> Product/1
  cos/1 -> Product1/1
  Low-Pass Filter (Discrete or Continuous)/1 -> We/1

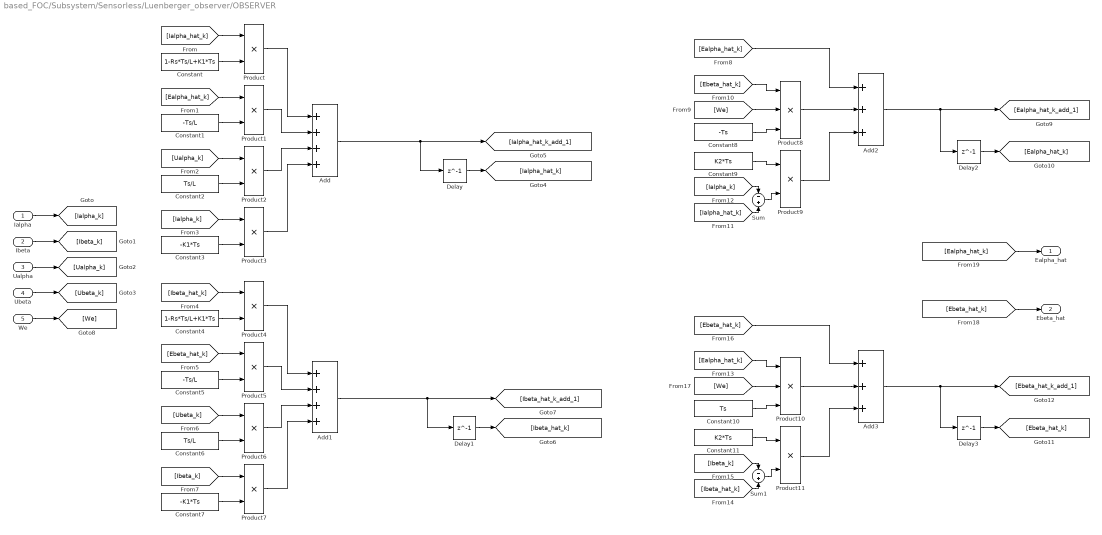
== system based_FOC/Subsystem/Sensorless/Luenberger_observer/OBSERVER ==
  Ialpha : Inport
  Ibeta : Inport  Port=2
  Ualpha : Inport  Port=3
  Ubeta : Inport  Port=4
  We : Inport  Port=5
  Add : Sum  Inputs=++++
  Add1 : Sum  Inputs=++++
  Add2 : Sum  Inputs=+++
  Add3 : Sum  Inputs=+++
  Constant : Constant  Value=1-Rs*Ts/L+K1*Ts
  Constant1 : Constant  Value=-Ts/L
  Constant10 : Constant  Value=Ts
  Constant11 : Constant  Value=K2*Ts
  Constant2 : Constant  Value=Ts/L
  Constant3 : Constant  Value=-K1*Ts
  Constant4 : Constant  Value=1-Rs*Ts/L+K1*Ts
  Constant5 : Constant  Value=-Ts/L
  Constant6 : Constant  Value=Ts/L
  Constant7 : Constant  Value=-K1*Ts
  Constant8 : Constant  Value=-Ts
  Constant9 : Constant  Value=K2*Ts
  Delay{,1..3} (4 alike) : Delay  DelayLength=1  InputProcessing=Columns as channels (frame based)
  Product{,1..7,9,11} (10 alike) : Product
  Product10 : Product  Inputs=3
  Product8 : Product  Inputs=3
  Sum : Sum  Inputs=-+
  Sum1 : Sum  Inputs=-+
  Ealpha_hat : Outport
  Ebeta_hat : Outport  Port=2
  wires:
  [Ialpha_hat_k] -> Product/1
  Constant/1 -> Product/2
  Product/1 -> Add/1
  [Ealpha_hat_k] -> Product1/1
  Constant1/1 -> Product1/2
  Constant2/1 -> Product2/2
  [Ualpha_k] -> Product2/1
  [Ialpha_k] -> Product3/1
  Constant3/1 -> Product3/2
  Product1/1 -> Add/2
  Product2/1 -> Add/3
  Product3/1 -> Add/4
  Ialpha/1 -> [Ialpha_k]
  Ubeta/1 -> [Ubeta_k]
  Ualpha/1 -> [Ualpha_k]
  Ibeta/1 -> [Ibeta_k]
  Delay/1 -> [Ialpha_hat_k]
  Delay1/1 -> [Ibeta_hat_k]
  [Ibeta_hat_k] -> Product4/1
  [Ibeta_k] -> Product7/1
  Constant7/1 -> Product7/2
  Constant5/1 -> Product5/2
  [Ebeta_hat_k] -> Product5/1
  Product6/1 -> Add1/3
  Product5/1 -> Add1/2
  [Ubeta_k] -> Product6/1
  Constant6/1 -> Product6/2
  Product7/1 -> Add1/4
  Constant4/1 -> Product4/2
  Product4/1 -> Add1/1
  We/1 -> [We]
  [We] -> Product8/2
  Constant8/1 -> Product8/3
  [Ebeta_hat_k] -> Product8/1
  [Ialpha_k] -> Sum/1
  [Ialpha_hat_k] -> Sum/2
  Constant9/1 -> Product9/1
  Sum/1 -> Product9/2
  Product9/1 -> Add2/3
  Delay2/1 -> [Ealpha_hat_k]
  [Ealpha_hat_k] -> Product10/1
  Constant10/1 -> Product10/3
  [Ebeta_hat_k] -> Add3/1
  [Ibeta_k] -> Sum1/1
  [We] -> Product10/2
  [Ibeta_hat_k] -> Sum1/2
  Delay3/1 -> [Ebeta_hat_k]
  Sum1/1 -> Product11/2
  Constant11/1 -> Product11/1
  Product11/1 -> Add3/3
  [Ealpha_hat_k] -> Ealpha_hat/1
  [Ebeta_hat_k] -> Ebeta_hat/1
  Product10/1 -> Add3/2
  Add/1 -> Delay/1, [Ialpha_hat_k_add_1]
  Add1/1 -> Delay1/1, [Ibeta_hat_k_add_1]
  Product8/1 -> Add2/2
  [Ealpha_hat_k] -> Add2/1
  Add3/1 -> Delay3/1, [Ebeta_hat_k_add_1]
  Add2/1 -> Delay2/1, [Ealpha_hat_k_add_1]

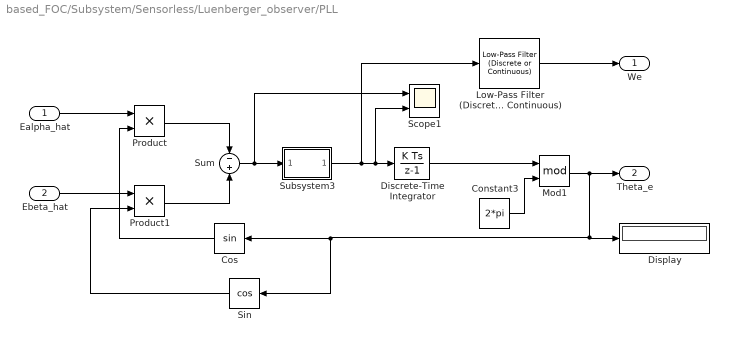
== system based_FOC/Subsystem/Sensorless/Luenberger_observer/PLL ==
  Ealpha_hat : Inport
  Ebeta_hat : Inport  Port=2
  Constant3 : Constant  Value=2*pi
  Cos : Trigonometry  NumberOfIterations=20
  Discrete-Time Integrator : DiscreteIntegrator  SampleTime=-1  ICPrevOutput=DiscIntNeverNeededParam  ICPrevScaledInput=DiscIntNeverNeededParam
  Display : Display
  Low-Pass Filter (Discrete or Continuous) : eeGeneralControl/Low-Pass Filter (Discrete or Continuous)  K=1  T=0.02  B=inf  A=-inf  init_option=Inherited from block input  x0=0  Ts=-1
  Mod1 : Math  Operator=mod
  Product : Product
  Product1 : Product
  Scope1 : Scope  NumInputPorts=2
  Sin : Trigonometry  Operator=cos  NumberOfIterations=20
  Subsystem3 : Subsystem  mask{Kp=35, Ki=10, Kd=0, Ts=0.0001, max_Integral=inf, min_Integral=-inf, max_output=inf, min_output=-inf}
      mask prompts: max_Integral "积分上限"; min_Integral "积分下限"; max_output "输出上限"; min_output "输出下限"
      mask DialogControl DescTextVar Prompt: PID控制器
      mask DialogControl ParameterGroupVar Prompt: 参数
      mask Display: fprintf('MyPID');
  Sum : Sum  Inputs=-+
  We : Outport
  Theta_e : Outport  Port=2
  wires:
  Mod1/1 -> Theta_e/1, Display/1, Sin/1, Cos/1
  Constant3/1 -> Mod1/2
  Subsystem3/1(output) -> Low-Pass Filter (Discrete or Continuous)/1, Scope1/2, Discrete-Time Integrator/1
  Sin/1 -> Product1/2
  Cos/1 -> Product/2
  Product/1 -> Sum/1
  Product1/1 -> Sum/2
  Discrete-Time Integrator/1 -> Mod1/1
  Sum/1 -> Subsystem3/1(error), Scope1/1
  Ebeta_hat/1 -> Product1/1
  Low-Pass Filter (Discrete or Continuous)/1 -> We/1
  Ealpha_hat/1 -> Product/1

== system based_FOC/Subsystem/Sensorless/Flux_observer/PLL/Subsystem3 ==
  error : Inport
  Constant : Constant  Value=Kp
  Constant1 : Constant  Value=Ki
  Constant2 : Constant  Value=Kd
  Constant3 : Constant  Value=Ts
  Constant4 : Constant  Value=max_Integral
  Constant5 : Constant  Value=min_Integral
  Constant6 : Constant  Value=max_output
  Constant7 : Constant  Value=min_output
  MATLAB Function : MATLAB Function  TreatAsAtomicUnit=on
  output : Outport
  wires:
  Constant3/1 -> MATLAB Function/5(Ts)
  Constant7/1 -> MATLAB Function/9(min_output)
  Constant/1 -> MATLAB Function/2(Kp)
  Constant4/1 -> MATLAB Function/6(max_Integral)
  Constant5/1 -> MATLAB Function/7(min_Integral)
  error/1 -> MATLAB Function/1(error)
  Constant1/1 -> MATLAB Function/3(Ki)
  Constant6/1 -> MATLAB Function/8(max_output)
  Constant2/1 -> MATLAB Function/4(Kd)
  MATLAB Function/1(output) -> output/1

== system based_FOC/Subsystem/Sensorless/Luenberger_observer/PLL/Subsystem3 ==
  error : Inport
  Constant : Constant  Value=Kp
  Constant1 : Constant  Value=Ki
  Constant2 : Constant  Value=Kd
  Constant3 : Constant  Value=Ts
  Constant4 : Constant  Value=max_Integral
  Constant5 : Constant  Value=min_Integral
  Constant6 : Constant  Value=max_output
  Constant7 : Constant  Value=min_output
  MATLAB Function : MATLAB Function  TreatAsAtomicUnit=on
  output : Outport
  wires:
  Constant3/1 -> MATLAB Function/5(Ts)
  Constant7/1 -> MATLAB Function/9(min_output)
  Constant/1 -> MATLAB Function/2(Kp)
  Constant4/1 -> MATLAB Function/6(max_Integral)
  Constant5/1 -> MATLAB Function/7(min_Integral)
  error/1 -> MATLAB Function/1(error)
  Constant1/1 -> MATLAB Function/3(Ki)
  Constant6/1 -> MATLAB Function/8(max_output)
  Constant2/1 -> MATLAB Function/4(Kd)
  MATLAB Function/1(output) -> output/1

== matlab function based_FOC/Subsystem/Sensorless/MATLAB Function ==
  data: U_alpha input; Tcm1 output; U_beta input; Period input; U_dc input; Tcm2 output; Tcm3 output
function [Tcm1, Tcm2, Tcm3] = fcn(U_alpha, U_beta, Period, U_dc)
    % 计算 Tx, Ty
    scaleFactor = -sqrt(3) * Period / 2 / U_dc;
    Tx = scaleFactor * (sqrt(3) * 0.5 * U_alpha + 0.5 * U_beta);
    Ty = scaleFactor * U_beta;

    % 计算 Ta, Tb, Tc
    if Tx >= 0 && Ty >= 0
        Tc = 0;
        [Ta, Tb] = myfun(Tx, Ty, Period);
    elseif Tx <= Ty && Tx <= 0
        Ta = 0;
        [Tb, Tc] = myfun(Ty - Tx, -Tx, Period);
    elseif Tx > Ty && Ty <= 0
        Tb = 0;
        [Ta, Tc] = myfun(Tx - Ty, -Ty, Period);
    else
        error('Both Tx and Ty cannot be less than 0');
    end

    % 计算 T0
    T_max = max([Ta, Tb, Tc]);
    T0 = Period / 2 - T_max;

    % 计算 Tcm1, Tcm2, Tcm3
    Tcm1 = Ta + T0 / 2;
    Tcm2 = Tb + T0 / 2;
    Tcm3 = Tc + T0 / 2;

    % Tcm2 = Ta + T0 / 2;
    % Tcm3 = Tb + T0 / 2;
    % Tcm1 = Tc + T0 / 2;
end

function [T1, T2] = myfun(T3, T4, Period)
    T3_abs = abs(T3);
    T4_abs = abs(T4);
    halfPeriod = Period / 2;

    if T3_abs <= halfPeriod && T4_abs <= halfPeriod
        T1 = T3;
        T2 = T4;
    elseif T3_abs >= halfPeriod && T4_abs >= halfPeriod
        T1 = halfPeriod;
        T2 = halfPeriod;
    elseif T3_abs >= T4_abs
        if T3_abs - T4_abs >= halfPeriod
            T1 = halfPeriod;
            T2 = 0;
        else
            T1 = halfPeriod;
            T2 = halfPeriod * T4 / T3;
        end
    else
        if T4_abs - T3_abs >= halfPeriod
            T1 = 0;
            T2 = halfPeriod;
        else
            T1 = halfPeriod * T3 / T4;
            T2 = halfPeriod;
        end
    end
end

== matlab function based_FOC/Subsystem/Sensorless/polarplot1 ==
  data: T_a input; T_b input; T_c input; U_alpha output; U_beta output
function [U_alpha ,U_beta] = fcn(T_a,T_b,T_c)
UA = T_a /4250*220;
UB = T_b /4250*220;
UC = T_c /4250*220;
U_alpha = UA -0.5*UB - 0.5*UC;
U_beta = (UB - UC)*sqrt(3)/2;
% R = sqrt(U_alpha^2+U_beta^2);
% theta = atan2d(U_beta,U_alpha);
end

== matlab function based_FOC/Subsystem/Sensorless/Anti_Park1/MATLAB Function ==
  data: Ualpha input; Ubeta input; y output; U_dc input
function y = fcn(Ualpha,Ubeta, U_dc)
    persistent count;
    u = sqrt(Ualpha^2 + Ubeta^2);
    % 设定阈值
    threshold = U_dc * 2 * sqrt(3) / 3;
    
    % 初始化 count
    if isempty(count)
        count = 0;
    end
    
    if count > 0
        % 若已触发，继续输出 1000 次
        y = threshold;
        count = count + 1;
        if count >= 1000
            count = 0; % 重置计数
        end
    else
        if u >= threshold
            count = 1; % 开始计数
            y = threshold;
        else
            y = u; % 正常计算输出
        end
    end
end

== matlab function based_FOC/Subsystem/Sensorless/Subsystem2/MATLAB Function ==
  data: error input; output output; Kp input; Ki input; Kd input; Ts input; max_Integral input; min_Integral input; max_output input; min_output input
function output = fcn(error, Kp, Ki, Kd, Ts, max_Integral, min_Integral, max_output, min_output)
%定义参数
persistent last_error;
persistent I;

% 初始化静态变量（仅在第一次调用时执行）
if isempty(last_error)
last_error = 0;  % 假设初始误差为0
end
if isempty(I)
I = 0;           % 假设初始积分项为0
end

%比例项
P = Kp*error;

%积分项
I = I + Ki*error*Ts;
%积分限幅
if(I>=max_Integral)
    I = max_Integral;
elseif(I<=min_Integral)
    I = min_Integral;
end

%微分项
D = Kd*(error - last_error)/Ts;

%保留此次错误值
last_error = error;

%输出限幅
output = P+I+D;
if(output>=max_output)
    output = max_output;
elseif(output<=min_output)
    output = min_output;
end

== matlab function based_FOC/Subsystem/Sensorless/Subsystem/MATLAB Function ==
  data: error input; output output; Kp input; Ki input; Kd input; Ts input; max_Integral input; min_Integral input; max_output input; min_output input
function output = fcn(error, Kp, Ki, Kd, Ts, max_Integral, min_Integral, max_output, min_output)
%定义参数
persistent last_error;
persistent I;

% 初始化静态变量（仅在第一次调用时执行）
if isempty(last_error)
last_error = 0;  % 假设初始误差为0
end
if isempty(I)
I = 0;           % 假设初始积分项为0
end

%比例项
P = Kp*error;

%积分项
I = I + Ki*error*Ts;
%积分限幅
if(I>=max_Integral)
    I = max_Integral;
elseif(I<=min_Integral)
    I = min_Integral;
end

%微分项
D = Kd*(error - last_error)/Ts;

%保留此次错误值
last_error = error;

%输出限幅
output = P+I+D;
if(output>=max_output)
    output = max_output;
elseif(output<=min_output)
    output = min_output;
end

== matlab function based_FOC/Subsystem/Sensorless/Subsystem3/MATLAB Function ==
  data: error input; output output; Kp input; Ki input; Kd input; Ts input; max_Integral input; min_Integral input; max_output input; min_output input
function output = fcn(error, Kp, Ki, Kd, Ts, max_Integral, min_Integral, max_output, min_output)
%定义参数
persistent last_error;
persistent I;

% 初始化静态变量（仅在第一次调用时执行）
if isempty(last_error)
last_error = 0;  % 假设初始误差为0
end
if isempty(I)
I = 0;           % 假设初始积分项为0
end

%比例项
P = Kp*error;

%积分项
I = I + Ki*error*Ts;
%积分限幅
if(I>=max_Integral)
    I = max_Integral;
elseif(I<=min_Integral)
    I = min_Integral;
end

%微分项
D = Kd*(error - last_error)/Ts;

%保留此次错误值
last_error = error;

%输出限幅
output = P+I+D;
if(output>=max_output)
    output = max_output;
elseif(output<=min_output)
    output = min_output;
end

== matlab function based_FOC/Subsystem/Sensorless/Flux_observer/PLL/Subsystem3/MATLAB Function ==
  data: error input; output output; Kp input; Ki input; Kd input; Ts input; max_Integral input; min_Integral input; max_output input; min_output input
function output = fcn(error, Kp, Ki, Kd, Ts, max_Integral, min_Integral, max_output, min_output)
%定义参数
persistent last_error;
persistent I;

% 初始化静态变量（仅在第一次调用时执行）
if isempty(last_error)
last_error = 0;  % 假设初始误差为0
end
if isempty(I)
I = 0;           % 假设初始积分项为0
end

%比例项
P = Kp*error;

%积分项
I = I + Ki*error*Ts;
%积分限幅
if(I>=max_Integral)
    I = max_Integral;
elseif(I<=min_Integral)
    I = min_Integral;
end

%微分项
D = Kd*(error - last_error)/Ts;

%保留此次错误值
last_error = error;

%输出限幅
output = P+I+D;
if(output>=max_output)
    output = max_output;
elseif(output<=min_output)
    output = min_output;
end

== matlab function based_FOC/Subsystem/Sensorless/Luenberger_observer/PLL/Subsystem3/MATLAB Function ==
  data: error input; output output; Kp input; Ki input; Kd input; Ts input; max_Integral input; min_Integral input; max_output input; min_output input
function output = fcn(error, Kp, Ki, Kd, Ts, max_Integral, min_Integral, max_output, min_output)
%定义参数
persistent last_error;
persistent I;

% 初始化静态变量（仅在第一次调用时执行）
if isempty(last_error)
last_error = 0;  % 假设初始误差为0
end
if isempty(I)
I = 0;           % 假设初始积分项为0
end

%比例项
P = Kp*error;

%积分项
I = I + Ki*error*Ts;
%积分限幅
if(I>=max_Integral)
    I = max_Integral;
elseif(I<=min_Integral)
    I = min_Integral;
end

%微分项
D = Kd*(error - last_error)/Ts;

%保留此次错误值
last_error = error;

%输出限幅
output = P+I+D;
if(output>=max_output)
    output = max_output;
elseif(output<=min_output)
    output = min_output;
end

== matlab function based_FOC/Subsystem/Sensorless/Subsystem1/MATLAB Function ==
  data: y output
function y = fcn()
persistent count;

% 初始化静态变量（仅在第一次调用时执行）
if isempty(count)
count = 1;  % 假设初始误差为0
end
%翻转电平
if(count == 1)
    count = -1;
elseif(count == -1)
    count = 1;
end

y = count*30;
